simulink library "librairie"  (Simulink 4.00)
libraries: cstblocks x1

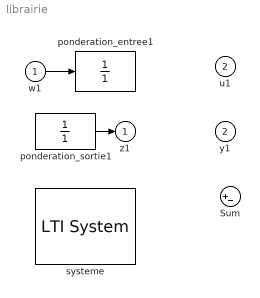
== system librairie ==
  w1 : Inport  Port=1  LatchInput=off
  u1 : Inport  Port=2  LatchInput=off
  Sum : Sum  Inputs=|+-  SaturateOnIntegerOverflow=on
  ponderation_entree1 : TransferFcn  Numerator=1  Denominator=1  AbsoluteTolerance=auto  Realization=auto
  ponderation_sortie1 : TransferFcn  Numerator=1  Denominator=1  AbsoluteTolerance=auto  Realization=auto
  systeme : cstblocks/LTI System  sys=tf(1)  IC=[]
  z1 : Outport  Port=1  InitialOutput=0
  y1 : Outport  Port=2  InitialOutput=0
  wires:
  ponderation_sortie1/1 -> z1/1
  w1/1 -> ponderation_entree1/1
